simulink model "DiscreteTD"  (R2018a)
settings: Solver=FixedStepAuto  StartTime=0.0  StopTime=20  FixedStep=0.01  RelTol=1e-3
settings Model: Creator=Administrator  LastModifiedBy=Administrator

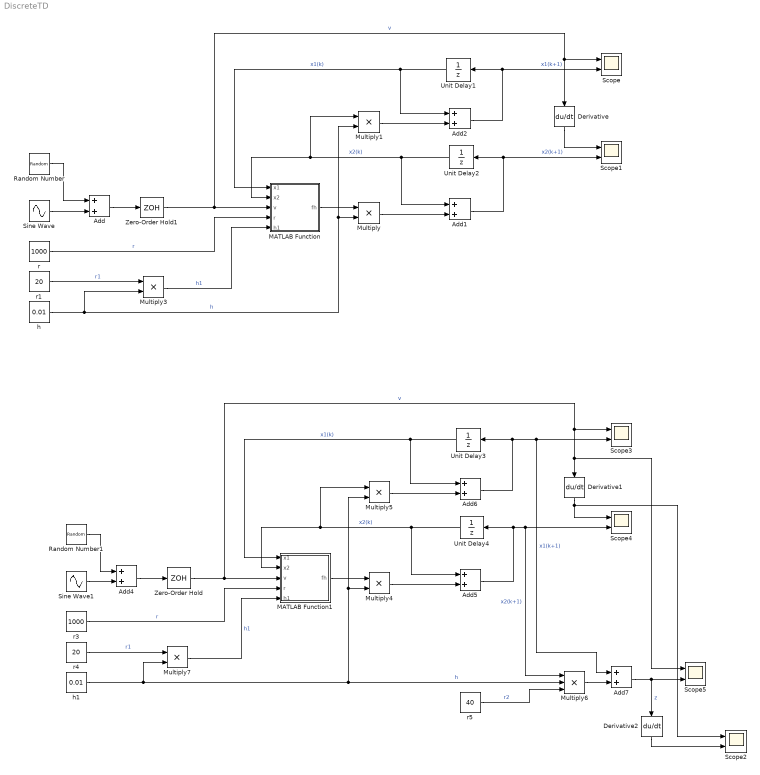
== system DiscreteTD ==
  Add{,1..2,4..7} (7 alike) : Sum
  Derivative : Derivative
  Derivative1 : Derivative
  Derivative2 : Derivative
  MATLAB Function : MATLAB Function  TreatAsAtomicUnit=on
  MATLAB Function1 : MATLAB Function  TreatAsAtomicUnit=on
  Multiply{,1,3..5,7} (6 alike) : Product
  Multiply6 : Product  Inputs=3
  Random Number : RandomNumber  Variance=0.1
  Random Number1 : RandomNumber  Variance=0.1
  Scope{,1..5} (6 alike) : Scope  NumInputPorts=2
  Sine Wave : Sin  Amplitude=2
  Sine Wave1 : Sin  Amplitude=2
  Unit Delay{1..4} (4 alike) : UnitDelay  SampleTime=-1
  Zero-Order Hold : ZeroOrderHold  SampleTime=-1
  Zero-Order Hold1 : ZeroOrderHold  SampleTime=-1
  h : Constant  Value=0.01
  h1 : Constant  Value=0.01
  r : Constant  Value=1000
  r1 : Constant  Value=20
  r3 : Constant  Value=1000
  r4 : Constant  Value=20
  r5 : Constant  Value=40
  wires:
  Sine Wave/1 -> Add/2
  Random Number/1 -> Add/1
  Multiply/1 -> Add1/2
  MATLAB Function/1(fh) -> Multiply/1
  Multiply1/1 -> Add2/2
  Unit Delay1/1 -> MATLAB Function/1(x1), Add2/1  "x1(k)"
  Add2/1 -> Unit Delay1/1, Scope/2  "x1(k+1)"
  Add1/1 -> Scope1/2, Unit Delay2/1  "x2(k+1)"
  Unit Delay2/1 -> Add1/1, Multiply1/1, MATLAB Function/2(x2)  "x2(k)"
  r/1 -> MATLAB Function/4(r)  "r"
  Add/1 -> Zero-Order Hold1/1
  Derivative/1 -> Scope1/1
  Multiply3/1 -> MATLAB Function/5(h1)  "h1"
  r1/1 -> Multiply3/1  "r1"
  h/1 -> Multiply1/2, Multiply/2, Multiply3/2  "h"
  Add5/1 -> Multiply6/1, Scope4/2, Unit Delay4/1  "x2(k+1)"
  Multiply7/1 -> MATLAB Function1/5(h1)  "h1"
  MATLAB Function1/1(fh) -> Multiply4/1
  Multiply6/1 -> Add7/2
  Add7/1 -> Scope5/2, Derivative2/1  "z"
  Sine Wave1/1 -> Add4/2
  Random Number1/1 -> Add4/1
  Unit Delay4/1 -> Add5/1, Multiply5/1, MATLAB Function1/2(x2)  "x2(k)"
  Multiply4/1 -> Add5/2
  h1/1 -> Multiply5/2, Multiply4/2, Multiply6/2, Multiply7/2  "h"
  Add6/1 -> Unit Delay3/1, Add7/1, Scope3/2  "x1(k+1)"
  r3/1 -> MATLAB Function1/4(r)  "r"
  Unit Delay3/1 -> MATLAB Function1/1(x1), Add6/1  "x1(k)"
  Multiply5/1 -> Add6/2
  Add4/1 -> Zero-Order Hold/1
  r4/1 -> Multiply7/1  "r1"
  Derivative1/1 -> Scope2/1, Scope4/1
  r5/1 -> Multiply6/3  "r2"
  Zero-Order Hold/1 -> Scope5/1, Derivative1/1, Scope3/1, MATLAB Function1/3(v)  "v"
  Zero-Order Hold1/1 -> Derivative/1, Scope/1, MATLAB Function/3(v)  "v"
  Derivative2/1 -> Scope2/2

== matlab function DiscreteTD/MATLAB Function1 ==
  data: x1 input; fh output; x2 input; v input; r input; h1 input
function fh = fhan(x1, x2, v, r, h1)
% h为滤波因子，r为调节系数，r越大跟踪效果越好，但微分信号会增加高颜噪声
% 反之，微分信号越平滑，会产生一定的滞后
d = r * h1;
d1 = h1 * r^2;
y = x1 - v + h1 * x2;
if (abs(y) >= d1)
    a = x2 + sign(y) * (sqrt(d^2+8*r*abs(y)) - d) / 2;
else
    a = x2 + y / h1;
end
fh = -r * sat(a, d);
end


function m = sat(a, d)
if (abs(a) >= d)
    m = sign(a);
else
    m = a / d;
end
end

== matlab function DiscreteTD/MATLAB Function ==
  data: x1 input; fh output; x2 input; v input; r input; h1 input
function fh = fhan(x1, x2, v, r, h1)
% h1为滤波因子，r为调节系数，r越大跟踪效果越好，但微分信号会增加高颜噪声
% 反之，微分信号越平滑，会产生一定的滞后
d = r * h1;
d1 = h1 * r^2;
y = x1 - v + h1 * x2;
if (abs(y) >= d1)
    a = x2 + sign(y) * (sqrt(d^2+8*r*abs(y)) - d) / 2;
else
    a = x2 + y / h1;
end
fh = -r * sat(a, d);
end

function m = sat(a, d)
if (abs(a) >= d)
    m = sign(a);
else
    m = a / d;
end
end
